simulink model "test_Hydrogen"  (R2021a)
settings: Solver=VariableStepAuto  StartTime=0.0  StopTime=10.0  RelTol=1e-3
values from neighbouring files (symbols this model uses):
  fuel_cell_power_rating = 50e6    (= 50000000)    [load_global_variables.m]
  H2_out_max = 150    [load_global_variables.m]
  H2_out_min = 0    [load_global_variables.m]
  Max_H2_P_Input = 260000000    [load_global_variables.m]
  Min_H2_P_Input = 1400    [load_global_variables.m]
  P_electrolysis_max = 570000    [load_global_variables.m]
  P_electrolysis_min = 0    [load_global_variables.m]
  Start_Tank_Fill_L = 1000    [load_global_variables.m]
settings Model: Creator=cm  LastModifiedBy=cm

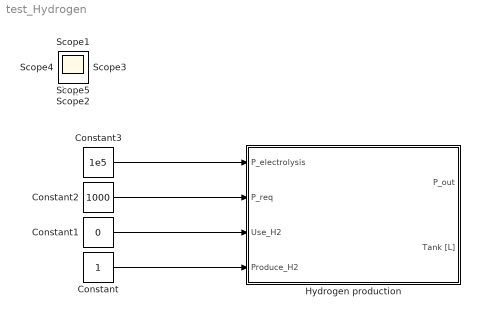
== system test_Hydrogen ==
  Constant : Constant
  Constant1 : Constant  Value=0
  Constant2 : Constant  Value=1000
  Constant3 : Constant  Value=1e5
  Hydrogen production : Subsystem
  Scope{,1..5} (6 alike) : Scope
  wires:
  Constant/1 -> Hydrogen production/4(Produce_H2)
  Constant1/1 -> Hydrogen production/3(Use_H2)
  Constant2/1 -> Hydrogen production/2(P_req)
  Constant3/1 -> Hydrogen production/1(P_electrolysis)

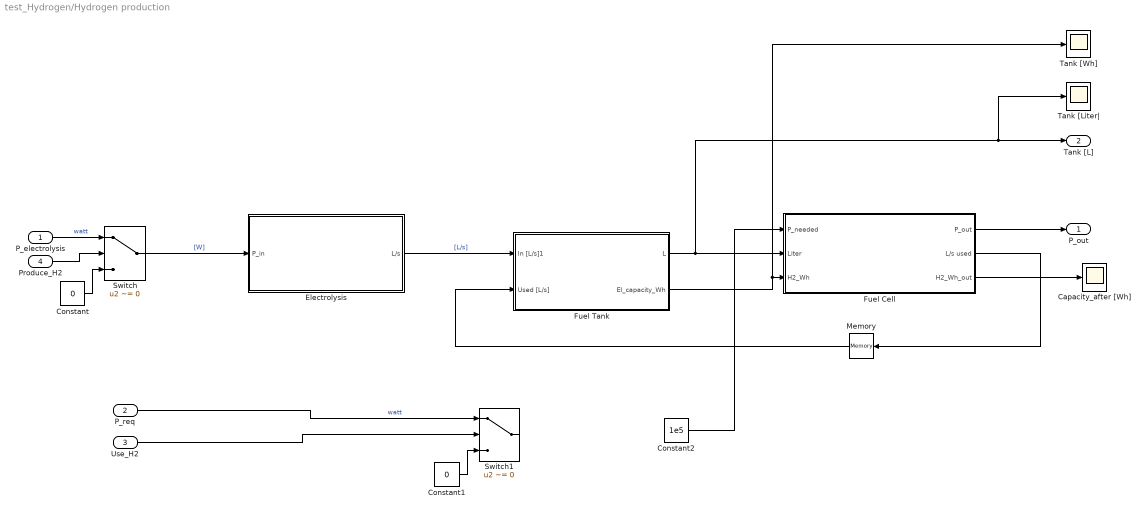
== system test_Hydrogen/Hydrogen production ==
  P_electrolysis : Inport
  P_req : Inport  Port=2
  Use_H2 : Inport  Port=3
  Produce_H2 : Inport  Port=4
  Capacity_after [Wh] : Scope
  Constant : Constant  Value=0
  Constant1 : Constant  Value=0
  Constant2 : Constant  Value=1e5
  Electrolysis : Subsystem
  Fuel Cell : Subsystem
  Fuel Tank : Subsystem
  Memory : Memory
  Switch : Switch  Criteria=u2 ~= 0  Threshold=1
  Switch1 : Switch  Criteria=u2 ~= 0  Threshold=1
  Tank [Liter| : Scope
  Tank [Wh] : Scope
  P_out : Outport
  Tank [L] : Outport  Port=2
  wires:
  Fuel Tank/1(L) -> Tank [Liter|/1, Tank [L]/1, Fuel Cell/2(Liter)
  Electrolysis/1(L/s) -> Fuel Tank/1(In [L/s]1)  "[L/s]"
  Fuel Cell/2(L/s used) -> Memory/1
  Fuel Cell/1(P_out) -> P_out/1
  Constant/1 -> Switch/3
  P_electrolysis/1 -> Switch/1  "watt"
  Constant1/1 -> Switch1/3
  P_req/1 -> Switch1/1  "watt"
  Produce_H2/1 -> Switch/2
  Use_H2/1 -> Switch1/2
  Memory/1 -> Fuel Tank/2(Used [L/s])
  Fuel Tank/2(El_capacity_Wh) -> Tank [Wh]/1, Fuel Cell/3(H2_Wh)
  Fuel Cell/3(H2_Wh_out) -> Capacity_after [Wh]/1
  Switch/1 -> Electrolysis/1(P_in)  "[W]"
  Constant2/1 -> Fuel Cell/1(P_needed)

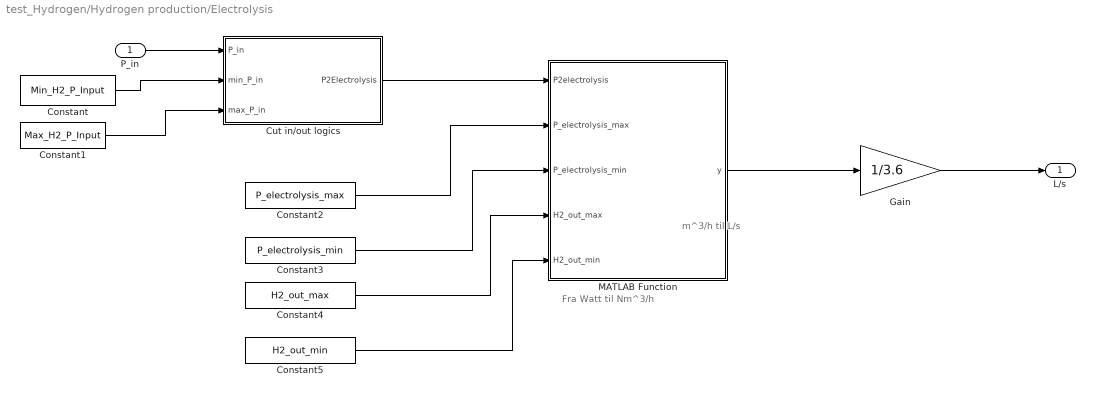
== system test_Hydrogen/Hydrogen production/Electrolysis ==
  note: m^3/h til L/s
  note: Fra Watt til Nm^3/h
  P_in : Inport
  Constant : Constant  Value=Min_H2_P_Input
  Constant1 : Constant  Value=Max_H2_P_Input
  Constant2 : Constant  Value=P_electrolysis_max
  Constant3 : Constant  Value=P_electrolysis_min
  Constant4 : Constant  Value=H2_out_max
  Constant5 : Constant  Value=H2_out_min
  Cut in/out logics : MATLAB Function  TreatAsAtomicUnit=on
  Gain : Gain  Gain=1/3.6
  MATLAB Function : MATLAB Function  TreatAsAtomicUnit=on
  L/s : Outport
  wires:
  P_in/1 -> Cut in/out logics/1(P_in)
  Constant/1 -> Cut in/out logics/2(min_P_in)
  Constant1/1 -> Cut in/out logics/3(max_P_in)
  Cut in/out logics/1(P2Electrolysis) -> MATLAB Function/1(P2electrolysis)
  MATLAB Function/1(y) -> Gain/1
  Gain/1 -> L/s/1
  Constant2/1 -> MATLAB Function/2(P_electrolysis_max)
  Constant3/1 -> MATLAB Function/3(P_electrolysis_min)
  Constant4/1 -> MATLAB Function/4(H2_out_max)
  Constant5/1 -> MATLAB Function/5(H2_out_min)

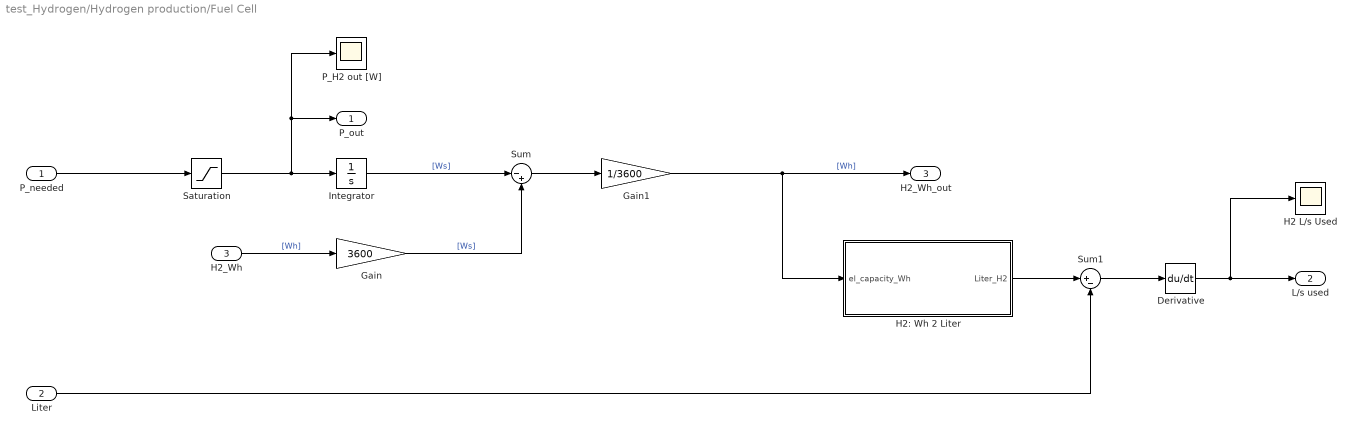
== system test_Hydrogen/Hydrogen production/Fuel Cell ==
  P_needed : Inport
  Liter : Inport  Port=2
  H2_Wh : Inport  Port=3
  Derivative : Derivative
  Gain : Gain  Gain=3600
  Gain1 : Gain  Gain=1/3600
  H2 L/s Used : Scope
  H2: Wh 2 Liter : MATLAB Function  TreatAsAtomicUnit=on
  Integrator : Integrator
  P_H2 out [W] : Scope
  Saturation : Saturate  UpperLimit=fuel_cell_power_rating  LowerLimit=0
  Sum : Sum  Inputs=|-+
  Sum1 : Sum  Inputs=|+-
  P_out : Outport
  L/s used : Outport  Port=2
  H2_Wh_out : Outport  Port=3
  wires:
  H2_Wh/1 -> Gain/1  "[Wh]"
  Integrator/1 -> Sum/1  "[Ws]"
  Gain/1 -> Sum/2  "[Ws]"
  Sum/1 -> Gain1/1
  Gain1/1 -> H2: Wh 2 Liter/1(el_capacity_Wh), H2_Wh_out/1  "[Wh]"
  P_needed/1 -> Saturation/1
  Saturation/1 -> P_H2 out [W]/1, P_out/1, Integrator/1
  Derivative/1 -> H2 L/s Used/1, L/s used/1
  H2: Wh 2 Liter/1(Liter_H2) -> Sum1/1
  Sum1/1 -> Derivative/1
  Liter/1 -> Sum1/2

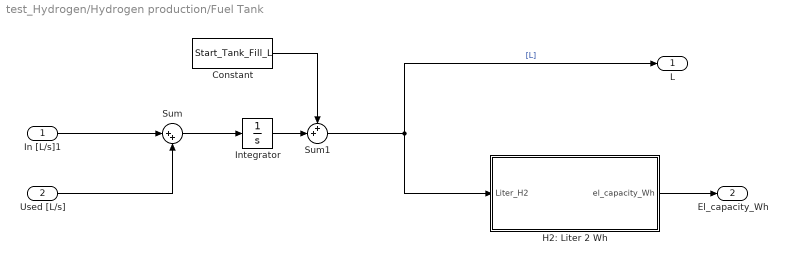
== system test_Hydrogen/Hydrogen production/Fuel Tank ==
  In [L/s]1 : Inport
  Used [L/s] : Inport  Port=2
  Constant : Constant  Value=Start_Tank_Fill_L
  H2: Liter 2 Wh : MATLAB Function  TreatAsAtomicUnit=on
  Integrator : Integrator
  Sum : Sum  Inputs=|++
  Sum1 : Sum  Inputs=++|
  L : Outport
  El_capacity_Wh : Outport  Port=2
  wires:
  Used [L/s]/1 -> Sum/2
  In [L/s]1/1 -> Sum/1
  Sum/1 -> Integrator/1
  Constant/1 -> Sum1/1
  Integrator/1 -> Sum1/2
  Sum1/1 -> H2: Liter 2 Wh/1(Liter_H2), L/1  "[L]"
  H2: Liter 2 Wh/1(el_capacity_Wh) -> El_capacity_Wh/1

== matlab function test_Hydrogen/Hydrogen production/Fuel Tank/H2: Liter 2 Wh ==
  data: Liter_H2 input; el_capacity_Wh output
function el_capacity_Wh = fcn(Liter_H2)

density_H2 = 42;  % [kg/m3]
potential_energy_H2 = 33.33e3; % [Wh/kg]; % [kg of hydrogen contains 33.33 kWh of usable energy]
% Pressurised hydrogen contains about 0.5 kWh/litre at 200 bar, 1.1 kWh/litre at 500 bar and 1.4 kWh/litre at 700 bar.

cubic_H2 = Liter_H2/1000; % [m^3]
el_capacity_Wh = potential_energy_H2*density_H2*cubic_H2;

== matlab function test_Hydrogen/Hydrogen production/Fuel Cell/H2: Wh 2 Liter ==
  data: el_capacity_Wh input; Liter_H2 output
function Liter_H2 = fcn(el_capacity_Wh)

density_H2 = 42;  % [kg/m3]
potential_energy_H2 = 33.33e3; % [Wh/kg]; % [kg of hydrogen contains 33.33 kWh of usable energy]


cubic_H2 = el_capacity_Wh/(potential_energy_H2*density_H2); % [m^3]

 Liter_H2 = cubic_H2*1000;

== matlab function test_Hydrogen/Hydrogen production/Electrolysis/Cut in//out logics ==
  data: P_in input; min_P_in input; P2Electrolysis output; max_P_in input
function P2Electrolysis = fcn(P_in, min_P_in, max_P_in)

if P_in >= min_P_in && P_in <= max_P_in
    
    P2Electrolysis = P_in;
elseif P_in > max_P_in
    P2Electrolysis = max_P_in;
elseif P_in < min_P_in
    P2Electrolysis = 0;
else
    % case shouldnt happen, but to secure our butts
    P2Electrolysis = max_P_in;
end

== matlab function test_Hydrogen/Hydrogen production/Electrolysis/MATLAB Function ==
  data: P2electrolysis input; P_electrolysis_max input; y output; P_electrolysis_min input; H2_out_max input; H2_out_min input
function y = fcn(P2electrolysis,P_electrolysis_max,P_electrolysis_min,H2_out_max, H2_out_min)
 
%Værdier for min og maks Elektrolyse 
% https://cellar-c2.services.clever-cloud.com/com-mcphy/uploads/2020/08/20.05.McPhy_Portfolio_ELY_Piel_EN.pdf

x2=P_electrolysis_max;
x1=P_electrolysis_min;

y2=H2_out_max;
y1=H2_out_min;


a=(y2-y1)/(x2-x1);

b=y1-a*x1;

y=a*P2electrolysis+b;
